simulink model "bumpem_control_system"  (R2021b)
settings: Solver=ode4  StartTime=0.0  StopTime=Inf  FixedStep=0.001  RelTol=1e-3
PostLoadFcn:
  | , if any(exist('dsrtsu_mdlpostloadfcn', 'file') == [2, 3, 6]), try dsrtsu_mdlpostloadfcn('Execute', bdroot); catch fprintf('Error in PostLoadFcn (dsrtsu_mdlpostloadfcn) for model "%s":\n %s\n', bdroot, lasterr); end, end,
libraries: rti1202lib_dac_class1 x4, simulink x4, dsparch4 x2, rti1202lib_adc_class1 x2
(part 2 of 2)

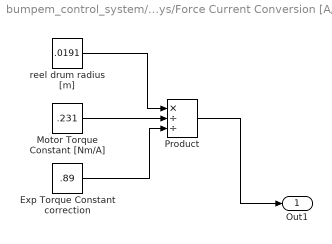
== system bumpem_control_system/Pertubration Subsys/Force Current Conversion [A//N] 1 ==
  Exp Torque Constant correction : Constant  Value=.89
  "Motor Torque Constant [Nm/A] " : Constant  Value=.231
  Product : Product  Inputs=*//
  "reel drum radius [m] " : Constant  Value=.0191
  Out1 : Outport  VectorParamsAs1DForOutWhenUnconnected=off
  wires:
  "Motor Torque Constant [Nm/A] "/1 -> Product/2
  Product/1 -> Out1/1
  "reel drum radius [m] "/1 -> Product/1
  Exp Torque Constant correction/1 -> Product/3

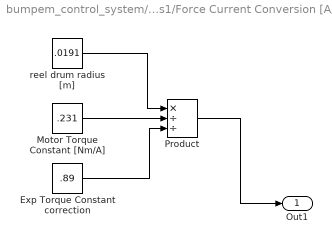
== system bumpem_control_system/Pertubration Subsys1/Force Current Conversion [A//N] 1 ==
  Exp Torque Constant correction : Constant  Value=.89
  "Motor Torque Constant [Nm/A] " : Constant  Value=.231
  Product : Product  Inputs=*//
  "reel drum radius [m] " : Constant  Value=.0191
  Out1 : Outport  VectorParamsAs1DForOutWhenUnconnected=off
  wires:
  "Motor Torque Constant [Nm/A] "/1 -> Product/2
  Product/1 -> Out1/1
  "reel drum radius [m] "/1 -> Product/1
  Exp Torque Constant correction/1 -> Product/3

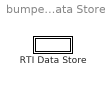
== system bumpem_control_system/RTI Data/RTI Data Store ==
  RTI Data Store : Subsystem  mask(RTI_DATA_STORE){}
      mask help:
      | RTI Data Store Block. This block is used by RTI to store internal model dependent data. Deleting this block will result in data loss.
      |
      | NEVER DELETE, COPY, OR MODIFY THIS BLOCK!
      mask Help:
      | RTI Data Store Block. This block is used by RTI to store internal model dependent data. Deleting this block will result in data loss.
      | 
      | NEVER DELETE, COPY, OR MODIFY THIS BLOCK!
      mask Display: text(0.5, 0.5, ' ', 'HorizontalAlignment', 'center');

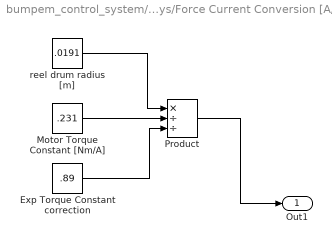
== system bumpem_control_system/Tracking Subsys/Force Current Conversion [A//N] 2 ==
  Exp Torque Constant correction : Constant  Value=.89
  "Motor Torque Constant [Nm/A] " : Constant  Value=.231
  Product : Product  Inputs=*//
  "reel drum radius [m] " : Constant  Value=.0191
  Out1 : Outport  VectorParamsAs1DForOutWhenUnconnected=off
  wires:
  "Motor Torque Constant [Nm/A] "/1 -> Product/2
  Product/1 -> Out1/1
  "reel drum radius [m] "/1 -> Product/1
  Exp Torque Constant correction/1 -> Product/3

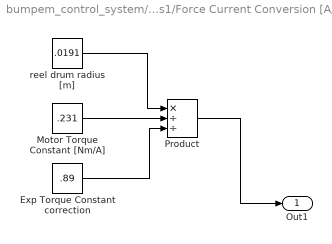
== system bumpem_control_system/Tracking Subsys1/Force Current Conversion [A//N] 2 ==
  Exp Torque Constant correction : Constant  Value=.89
  "Motor Torque Constant [Nm/A] " : Constant  Value=.231
  Product : Product  Inputs=*//
  "reel drum radius [m] " : Constant  Value=.0191
  Out1 : Outport  VectorParamsAs1DForOutWhenUnconnected=off
  wires:
  "Motor Torque Constant [Nm/A] "/1 -> Product/2
  Product/1 -> Out1/1
  "reel drum radius [m] "/1 -> Product/1
  Exp Torque Constant correction/1 -> Product/3

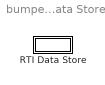
== system bumpem_control_system/RTI Data/RTI Data Store/RTI Data Store ==
  RTI Data Store : Subsystem  mask(RTI_DATA_STORE){}
      mask help:
      | RTI Data Store Block. This block is used by RTI to store internal model dependent data. Deleting this block will result in data loss.
      |
      | NEVER DELETE, COPY, OR MODIFY THIS BLOCK!
      mask Help:
      | RTI Data Store Block. This block is used by RTI to store internal model dependent data. Deleting this block will result in data loss.
      | 
      | NEVER DELETE, COPY, OR MODIFY THIS BLOCK!
      mask Display: text(0.5, 0.5, ' ', 'HorizontalAlignment', 'center');

== system bumpem_control_system/RTI Data/RTI Data Store/RTI Data Store/RTI Data Store ==
  RTI Data Store : Subsystem  mask(RTI_DATA_STORE){}
      mask help:
      | RTI Data Store Block. This block is used by RTI to store internal model dependent data. Deleting this block will result in data loss.
      |
      | NEVER DELETE, COPY, OR MODIFY THIS BLOCK!
      mask Help:
      | RTI Data Store Block. This block is used by RTI to store internal model dependent data. Deleting this block will result in data loss.
      | 
      | NEVER DELETE, COPY, OR MODIFY THIS BLOCK!
      mask Display: text(0.5, 0.5, ' ', 'HorizontalAlignment', 'center');

== system bumpem_control_system/RTI Data/RTI Data Store/RTI Data Store/RTI Data Store/RTI Data Store ==
